simulink model "DC_MOTOR"  (R2020b)
settings: Solver=VariableStepAuto  StartTime=0.0  StopTime=10.0  RelTol=1e-3
settings Model: Creator=SWARUP  LastModifiedBy=SWARUP

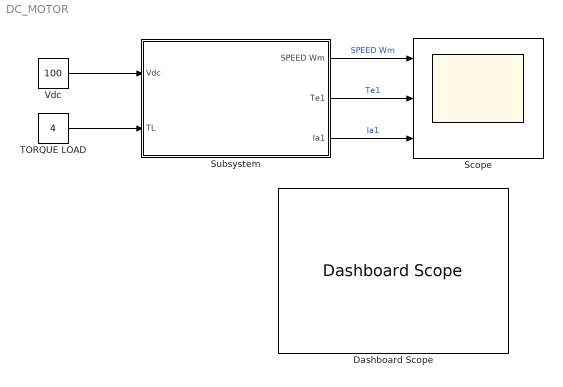
== system DC_MOTOR ==
  Dashboard Scope : DashboardScope
  Scope : Scope  NumInputPorts=3
  Subsystem : Subsystem
  TORQUE LOAD : Constant  Value=4
  Vdc : Constant  Value=100
  wires:
  Vdc/1 -> Subsystem/1(Vdc)
  TORQUE LOAD/1 -> Subsystem/2(TL)
  Subsystem/1(SPEED Wm) -> Scope/1  "SPEED Wm"
  Subsystem/2(Te1) -> Scope/2  "Te1"
  Subsystem/3(Ia1) -> Scope/3  "Ia1"

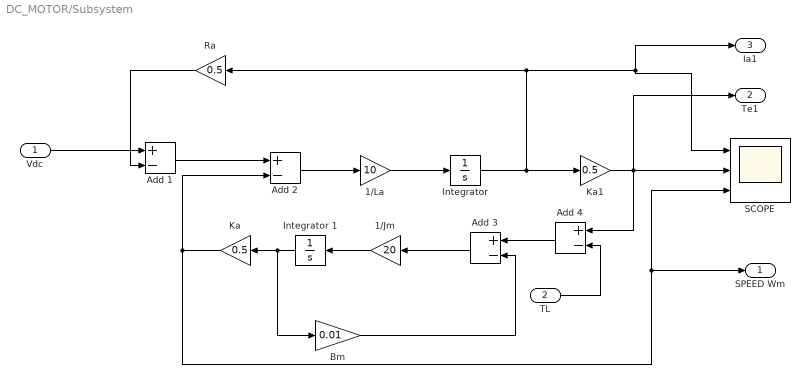
== system DC_MOTOR/Subsystem ==
  Vdc : Inport
  TL : Inport  Port=2
  1/Jm : Gain  Gain=20
  1/La : Gain  Gain=10
  Add {1..4} (4 alike) : Sum  Inputs=+-
  Bm : Gain  Gain=0.01
  "Integrator " : Integrator
  Integrator 1 : Integrator
  Ka : Gain  Gain=0.5
  Ka1 : Gain  Gain=0.5
  Ra : Gain  Gain=0.5
  SCOPE : Scope  NumInputPorts=3
  SPEED Wm : Outport
  Te1 : Outport  Port=2
  Ia1 : Outport  Port=3
  wires:
  "Integrator "/1 -> Ia1/1, SCOPE/1, Ra/1, Ka1/1
  Ra/1 -> Add 1/2
  Ka1/1 -> Te1/1, SCOPE/2, Add 4/1
  Add 1/1 -> Add 2/1
  Ka/1 -> Add 2/2, SPEED Wm/1, SCOPE/3
  TL/1 -> Add 4/2
  Bm/1 -> Add 3/2
  Add 3/1 -> 1/Jm/1
  Integrator 1/1 -> Bm/1, Ka/1
  1/La/1 -> "Integrator "/1
  Add 4/1 -> Add 3/1
  1/Jm/1 -> Integrator 1/1
  Vdc/1 -> Add 1/1
  Add 2/1 -> 1/La/1
